simulink model "UDP_simulink"  (R2020b)
settings: Solver=FixedStepAuto  StartTime=0.0  StopTime=50  FixedStep=0.001  RelTol=1e-3
libraries: etargetslib x1, dspnetwork x1
settings Model: EnablePacing=on  Creator=simon  LastModifiedBy=simon

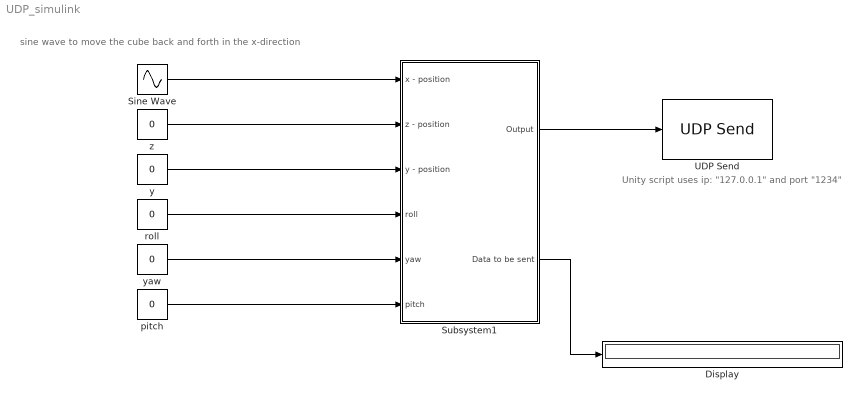
== system UDP_simulink ==
  note: sine wave to move the cube back and forth in the x-direction
  note: Unity script uses ip: "127.0.0.1" and port "1234"
  Display : Display
  Sine Wave : Sin  Amplitude=5  SampleTime=0.001
  Subsystem1 : Subsystem
  UDP Send : dspnetwork/UDP Send  remoteURL='127.0.0.1'  remotePort=1234  localURL='0.0.0.0'  localPortSource=Automatically determine  localPort=-1  sendBufferSize=8192  sampletime=-1  blockPlatform=HOST  separateLengthPort=0
  pitch : Constant  Value=0
  roll : Constant  Value=0
  y : Constant  Value=0
  yaw : Constant  Value=0
  z : Constant  Value=0
  wires:
  z/1 -> Subsystem1/2(z - position)
  Subsystem1/1(Output) -> UDP Send/1
  Sine Wave/1 -> Subsystem1/1(x - position)
  Subsystem1/2(Data to be sent) -> Display/1
  y/1 -> Subsystem1/3(y - position)
  roll/1 -> Subsystem1/4(roll)
  yaw/1 -> Subsystem1/5(yaw)
  pitch/1 -> Subsystem1/6(pitch)

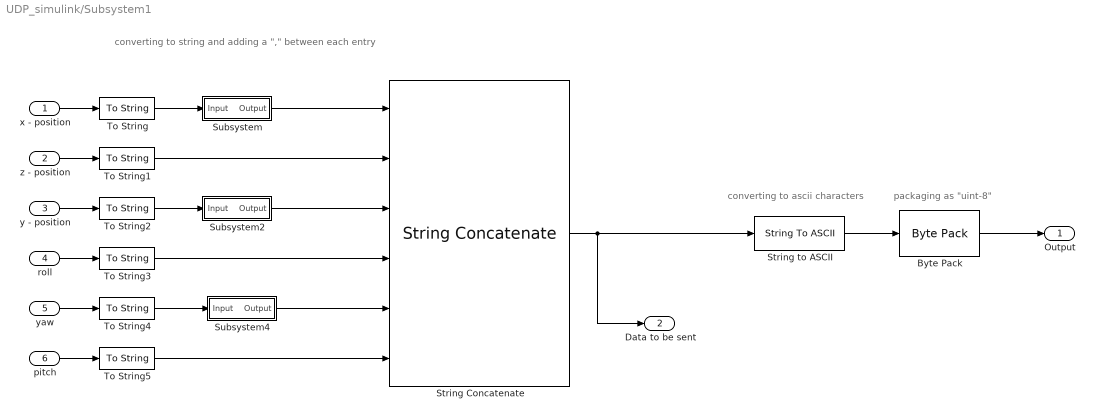
== system UDP_simulink/Subsystem1 ==
  note: packaging as "uint-8"
  note: converting to ascii characters
  note: converting to string and adding a "," between each entry
  x - position : Inport
  z - position : Inport  Port=2
  y - position : Inport  Port=3
  roll : Inport  Port=4
  yaw : Inport  Port=5
  pitch : Inport  Port=6
  Byte Pack : etargetslib/Byte Pack  datatypes={'uint8'}  byteAlign=1
  String Concatenate : StringConcatenate  Inputs=6
  String to ASCII : StringToASCII  OutputVectorSize=64
  Subsystem : Subsystem
  Subsystem2 : Subsystem
  Subsystem4 : Subsystem
  To String{,1..5} (6 alike) : ToString
  Output : Outport
  Data to be sent : Outport  Port=2
  wires:
  String Concatenate/1 -> Data to be sent/1, String to ASCII/1
  To String3/1 -> String Concatenate/4
  To String2/1 -> Subsystem2/1(Input)
  Subsystem4/1(Output) -> String Concatenate/5
  String to ASCII/1 -> Byte Pack/1
  To String/1 -> Subsystem/1(Input)
  To String5/1 -> String Concatenate/6
  Subsystem2/1(Output) -> String Concatenate/3
  To String1/1 -> String Concatenate/2
  To String4/1 -> Subsystem4/1(Input)
  Subsystem/1(Output) -> String Concatenate/1
  Byte Pack/1 -> Output/1
  z - position/1 -> To String1/1
  x - position/1 -> To String/1
  pitch/1 -> To String5/1
  roll/1 -> To String3/1
  yaw/1 -> To String4/1
  y - position/1 -> To String2/1

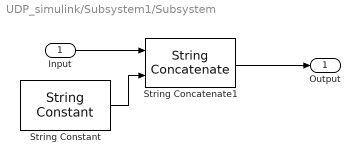
== system UDP_simulink/Subsystem1/Subsystem ==
  Input : Inport
  String Concatenate1 : StringConcatenate
  String Constant : StringConstant  String="\",\""
  Output : Outport
  wires:
  Input/1 -> String Concatenate1/1
  String Constant/1 -> String Concatenate1/2
  String Concatenate1/1 -> Output/1

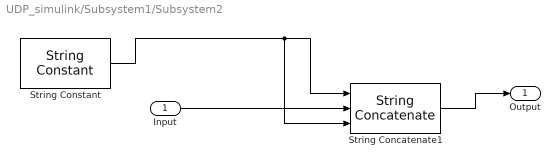
== system UDP_simulink/Subsystem1/Subsystem2 ==
  Input : Inport
  String Concatenate1 : StringConcatenate  Inputs=3
  String Constant : StringConstant  String="\",\""
  Output : Outport
  wires:
  String Concatenate1/1 -> Output/1
  Input/1 -> String Concatenate1/2
  String Constant/1 -> String Concatenate1/3, String Concatenate1/1

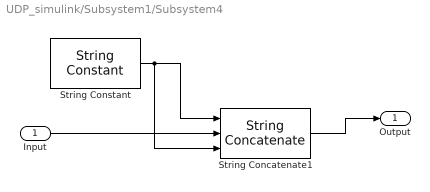
== system UDP_simulink/Subsystem1/Subsystem4 ==
  Input : Inport
  String Concatenate1 : StringConcatenate  Inputs=3
  String Constant : StringConstant  String="\",\""
  Output : Outport
  wires:
  String Concatenate1/1 -> Output/1
  Input/1 -> String Concatenate1/2
  String Constant/1 -> String Concatenate1/3, String Concatenate1/1
